simulink subsystem "window_taper"  (R2019b)
settings: Solver=VariableStepAuto  StartTime=0.0  StopTime=10.0  RelTol=1e-3
model mask{windowFun=taylorwin(128,10,-40)}
  mask prompts: windowFun "Window Function"
settings Model: Creator=gua0154  LastModifiedBy=gua0154

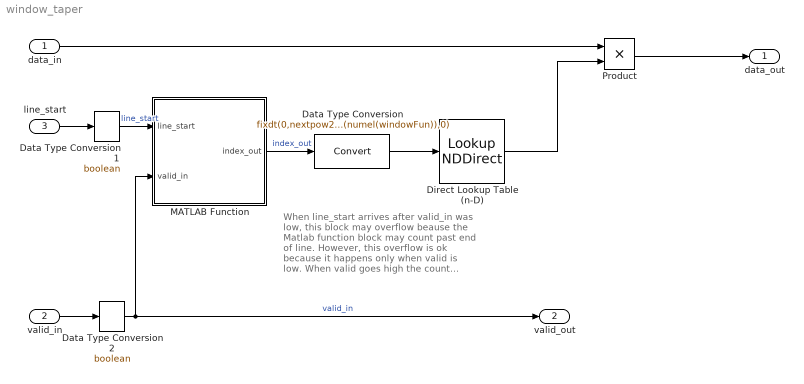
== system window_taper ==
  note: When line_start arrives after valid_in was low, this block may overflow beause the Matlab function block may count past end of line. However, this overflow is ok because it happens only when valid is low. When valid goes high the count resets to zero automatically
  data_in : Inport
  valid_in : Inport  Port=2
  line_start : Inport  Port=3
  Data Type Conversion : DataTypeConversion  OutDataTypeStr=fixdt(0,nextpow2(numel(windowFun)),0)
  Data Type Conversion1 : DataTypeConversion  OutDataTypeStr=boolean
  Data Type Conversion2 : DataTypeConversion  OutDataTypeStr=boolean
  Direct Lookup Table (n-D) : LookupNDDirect  NumberOfTableDimensions=1  Table=windowFun  DiagnosticForOutOfRangeInput=Error
  MATLAB Function : MATLAB Function  TreatAsAtomicUnit=on
  Product : Product
  data_out : Outport
  valid_out : Outport  Port=2
  wires:
  Product/1 -> data_out/1
  data_in/1 -> Product/1
  Direct Lookup Table (n-D)/1 -> Product/2
  valid_in/1 -> Data Type Conversion2/1
  MATLAB Function/1(index_out) -> Data Type Conversion/1  "index_out"
  line_start/1 -> Data Type Conversion1/1
  Data Type Conversion/1 -> Direct Lookup Table (n-D)/1
  Data Type Conversion1/1 -> MATLAB Function/1(line_start)  "line_start"
  Data Type Conversion2/1 -> MATLAB Function/2(valid_in), valid_out/1  "valid_in"

== matlab function window_taper/MATLAB Function ==
  data: line_start input; index_out output; valid_in input
function index_out = fcn(line_start,valid_in)
% compute index into the lookup table
% start at zero when we see line_start go high

% address length for the counter
ADDR_LENGTH = 32;

persistent count
if isempty(count)
    count = fi(0,0,ADDR_LENGTH,0);
end

if line_start 
    % if we see line_start go high, reset the counter
    count = fi(0,0,ADDR_LENGTH,0);
end

% count for the current clock
index_out = count;

% compute for the next clock
if valid_in
    % advance to the next index
    count = fi(count + 1,0,ADDR_LENGTH,0);
end
